simulink model "PID_PositionControl_SL"  (R2017b)
settings: Solver=VariableStepAuto  StartTime=0.0  StopTime=100  RelTol=1e-3
values from neighbouring files (symbols this model uses):
  Kd = 0    [ForceController.m]    (also in ForceController_Stabilization.m; PID_PositionControl.m; PositionController.m; StateMachine.m)
  Ki = 2    [ForceController.m]    (also in ForceController_Stabilization.m = 3; PID_PositionControl.m; PositionController.m; StateMachine.m = 3)
  Kp = 15    [ForceController.m]    (also in ForceController_Stabilization.m = 20; PID_PositionControl.m; PositionController.m; StateMachine.m)
libraries: checkpacklib x2, simulink x1
settings Model: Creator=Guillermo Herrera  LastModifiedBy=Guillermo Herrera

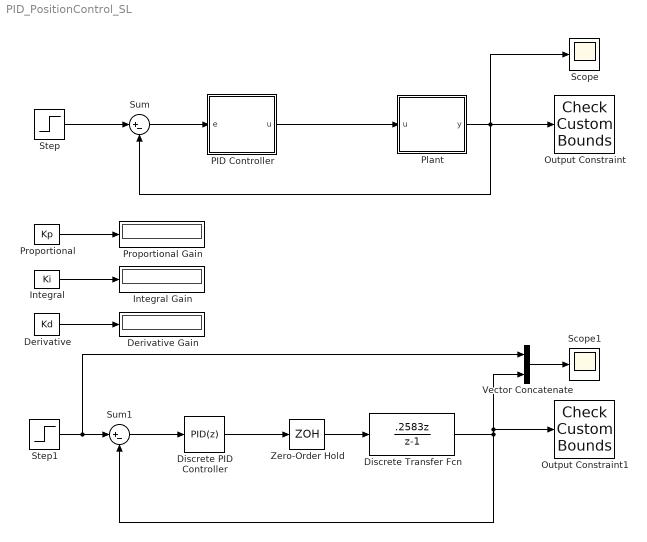
== system PID_PositionControl_SL ==
  Derivative : Constant  Value=Kd
  Derivative Gain : Display
  Discrete Transfer Fcn : DiscreteTransferFcn  Numerator=[.2583 0]  Denominator=[1 -1]
  Discrete PID Controller : simulink/Continuous/PID Controller  Controller=PID  TimeDomain=Discrete-time  SampleTime=-1  IntegratorMethod=Forward Euler  FilterMethod=Forward Euler  Form=Parallel  UseFilter=on  ControllerParametersSource=internal  P=1  I=1  D=1  N=100  InitialConditionSource=internal  InitialConditionForIntegrator=0  InitialConditionForFilter=0  ExternalReset=none  LimitOutput=off  UpperSaturationLimit=inf  LowerSaturationLimit=-inf  LinearizeAsGain=off  AntiWindupMode=none  Kb=1  TrackingMode=off  Kt=1  PParamMin=[]  PParamMax=[]  IParamMin=[]  IParamMax=[]  DParamMin=[]  DParamMax=[]  NParamMin=[]  NParamMax=[]  KbParamMin=[]  KbParamMax=[]  KtParamMin=[]  KtParamMax=[]  POutMin=[]  POutMax=[]  IOutMin=[]  IOutMax=[]  DOutMin=[]  DOutMax=[]  NOutMin=[]  NOutMax=[]  KbOutMin=[]  KbOutMax=[]  KtOutMin=[]  KtOutMax=[]  IntegratorOutMin=[]  IntegratorOutMax=[]  FilterOutMin=[]  FilterOutMax=[]  SumOutMin=[]  SumOutMax=[]  SumI1OutMin=[]  SumI1OutMax=[]  SumI2OutMin=[]  SumI2OutMax=[]  SumI3OutMin=[]  SumI3OutMax=[]  SumDOutMin=[]  SumDOutMax=[]  SaturationOutMin=[]  SaturationOutMax=[]  IntegratorContinuousStateAttributes=''  IntegratorStateMustResolveToSignalObject=off  IntegratorRTWStateStorageClass=Auto  FilterContinuousStateAttributes=''  FilterStateMustResolveToSignalObject=off  FilterRTWStateStorageClass=Auto  DifferentiatorICPrevScaledInput=0  DifferentiatorOutMin=[]  DifferentiatorOutMax=[]  InitialConditionSetting=State (most efficient)  FilterDiffOutCoefMin=[]  FilterDiffOutCoefMax=[]  SumDenOutMin=[]  SumDenOutMax=[]  SumNumOutMin=[]  SumNumOutMax=[]  ReciprocalOutMin=[]  ReciprocalOutMax=[]  DivideOutMin=[]  DivideOutMax=[]  TunerSelectOption=Transfer Function Based (PID Tuner App)
  Integral : Constant  Value=Ki
  Integral Gain : Display
  Output Constraint : checkpacklib/Check Custom Bounds  InstantiateOnLoad=on  enabled=on  stopWhenAssertionFail=off  export=off  ViewDlgPos=[1 41 1280 607.333333333333]  OpenViewOnLoad=off  LaunchViewOnOpen=on  TimeUnits=seconds  EnableUpperBound=on  UpperBoundTimes=[0 3;3 4.5;4.5 Inf]  UpperBoundAmplitudes=[0.44 0.44;0.42 0.42;0.42 0.42]  EnableLowerBound=on  LowerBoundTimes=[0 2;2 3;3 4.5;4.5 Inf]  LowerBoundAmplitudes=[-0.04 -0.04;0.32 0.32;0.38 0.38;0.38 0.38]
  Output Constraint1 : checkpacklib/Check Custom Bounds  InstantiateOnLoad=on  enabled=on  stopWhenAssertionFail=off  export=off  ViewDlgPos=[1 41 1280 607.333333333333]  OpenViewOnLoad=off  LaunchViewOnOpen=on  TimeUnits=seconds  EnableUpperBound=on  UpperBoundTimes=[0 10;10 15;15 Inf]  UpperBoundAmplitudes=[1.65 1.65;1.575 1.575;1.575 1.575]  EnableLowerBound=on  LowerBoundTimes=[0 5;5 10;10 15;15 Inf]  LowerBoundAmplitudes=[-0.15 -0.15;1.2 1.2;1.425 1.425;1.425 1.425]
  PID Controller : Subsystem
  Plant : Subsystem
  Proportional : Constant  Value=Kp
  Proportional Gain : Display
  Scope : Scope
  Scope1 : Scope
  Step : Step  After=1.5  SampleTime=.0338
  Step1 : Step  After=1.5  SampleTime=.0338
  Sum : Sum  Inputs=|+-
  Sum1 : Sum  Inputs=|+-
  Vector Concatenate : Concatenate
  Zero-Order Hold : ZeroOrderHold  SampleTime=-1
  wires:
  Step/1 -> Sum/1
  Proportional/1 -> Proportional Gain/1
  Integral/1 -> Integral Gain/1
  Derivative/1 -> Derivative Gain/1
  Plant/1(y) -> Scope/1, Sum/2, Output Constraint/1
  Sum/1 -> PID Controller/1(e)
  PID Controller/1(u) -> Plant/1("u ")
  Step1/1 -> Vector Concatenate/1, Sum1/1
  Zero-Order Hold/1 -> Discrete Transfer Fcn/1
  Discrete Transfer Fcn/1 -> Vector Concatenate/2, Output Constraint1/1, Sum1/2
  Vector Concatenate/1 -> Scope1/1
  Discrete PID Controller/1 -> Zero-Order Hold/1
  Sum1/1 -> Discrete PID Controller/1

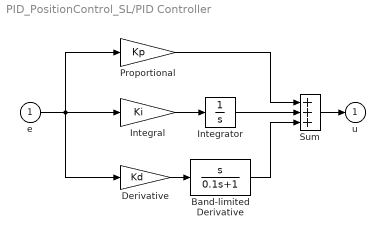
== system PID_PositionControl_SL/PID Controller ==
  e : Inport
  Band-limited Derivative : TransferFcn  Numerator=[1 0]  Denominator=[0.1 1]
  Derivative : Gain  Gain=Kd  SaturateOnIntegerOverflow=on  OutDataTypeStr=Inherit: Same as input  ParamDataTypeStr=Inherit: Same as input
  Integral : Gain  Gain=Ki  SaturateOnIntegerOverflow=on  OutDataTypeStr=Inherit: Same as input  ParamDataTypeStr=Inherit: Same as input
  Integrator : Integrator
  Proportional : Gain  Gain=Kp  SaturateOnIntegerOverflow=on  OutDataTypeStr=Inherit: Same as input  ParamDataTypeStr=Inherit: Same as input
  Sum : Sum  Inputs=+++  SaturateOnIntegerOverflow=on  InputSameDT=on  OutDataTypeStr=Inherit: Same as first input
  u : Outport  InitialOutput=0
  wires:
  Proportional/1 -> Sum/1
  Integral/1 -> Integrator/1
  Band-limited Derivative/1 -> Sum/3
  e/1 -> Integral/1, Proportional/1, Derivative/1
  Sum/1 -> u/1
  Derivative/1 -> Band-limited Derivative/1
  Integrator/1 -> Sum/2

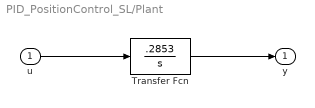
== system PID_PositionControl_SL/Plant ==
  "u " : Inport
  Transfer Fcn : TransferFcn  Numerator=[.2853]  Denominator=[1 0]
  y : Outport  InitialOutput=0
  wires:
  Transfer Fcn/1 -> y/1
  "u "/1 -> Transfer Fcn/1
